simulink model "pfb_coeff_sim"  (R2016b)
settings: Solver=VariableStepAuto  StartTime=0.0  StopTime=8192*0.5  RelTol=1e-3
undefined symbols (not defined in the file): fft_stages
libraries: xbsIndex_r4 x6420, casper_library_misc x5, casper_library_sources x4, xps_library x1, casper_library_delays x1
(part 6 of 36)

== system pfb_coeff_sim/pfb ==
  note: Controls whether there is
      | a shift to the right after
      | multiplication at the
      | respective stage in the
      | fft to prevent
      | overflow.
  note: polyphase FIR and FFT
  shift : Inport
  sync_in : Inport  Port=2
  din0 : Inport  Port=3
  din1 : Inport  Port=4
  en : Inport  Port=5
  Constant : xbsIndex_r4/Constant  const=0  gui_display_data_type=Boolean  arith_type=Boolean  n_bits=16  bin_pt=14  preci_type=Single  exp_width=8  frac_width=24  explicit_period=on  period=1  equ=P=C  opselect=C  inp2=PCIN>>17  opr=+  inp1=P  carry=CIN  dbl_ovrd=off  block_type=constant
  Constant1 : xbsIndex_r4/Constant  const=0  gui_display_data_type=Boolean  arith_type=Boolean  n_bits=16  bin_pt=14  preci_type=Single  exp_width=8  frac_width=24  explicit_period=on  period=1  equ=P=C  opselect=C  inp2=PCIN>>17  opr=+  inp1=P  carry=CIN  dbl_ovrd=off  block_type=constant
  Constant2 : xbsIndex_r4/Constant  const=0  gui_display_data_type=Fixed-point  arith_type=Signed (2's comp)  n_bits=18  bin_pt=17  preci_type=Single  exp_width=8  frac_width=24  explicit_period=on  period=1  equ=P=C  opselect=C  inp2=PCIN>>17  opr=+  inp1=P  carry=CIN  dbl_ovrd=off  block_type=constant
  Constant3 : xbsIndex_r4/Constant  const=0  gui_display_data_type=Fixed-point  arith_type=Unsigned  n_bits=4  bin_pt=0  preci_type=Single  exp_width=8  frac_width=24  explicit_period=on  period=1  equ=P=C  opselect=C  inp2=PCIN>>17  opr=+  inp1=P  carry=CIN  dbl_ovrd=off  block_type=constant
  Constant34 : xbsIndex_r4/Constant  const=0  gui_display_data_type=Fixed-point  arith_type=Unsigned  n_bits=2  bin_pt=0  preci_type=Single  exp_width=8  frac_width=24  explicit_period=on  period=1  equ=P=C  opselect=C  inp2=PCIN>>17  opr=+  inp1=P  carry=CIN  dbl_ovrd=off  block_type=constant
  Gateway Out{1..7,16..17,19,53} (11 alike) : xbsIndex_r4/Gateway Out  inherit_from_input=off  hdl_port=off  rows=1  columns=1  UseAsDAC=off  DACChannel='1'  interface=None  automatic_assignment=on  address_offset=hex2dec('00')  intf_name=''  intf_description=''  timing_constraint=None  locs_specified=off  LOCs={}  io_standard={}  block_type=gatewayout
  Terminator{1..9} (9 alike) : Terminator
  To Workspace16 : ToWorkspace  VariableName=fir_sync_in  SaveFormat=Timeseries  SampleTime=-1
  To Workspace17 : ToWorkspace  VariableName=fir_sync_out  SaveFormat=Timeseries  SampleTime=-1
  To Workspace19 : ToWorkspace  VariableName=fir_dv  SaveFormat=Timeseries  SampleTime=-1
  To Workspace2 : ToWorkspace  VariableName=fir1  SaveFormat=Timeseries  SampleTime=-1
  To Workspace3 : ToWorkspace  VariableName=fir2  SaveFormat=Timeseries  SampleTime=-1
  To Workspace4 : ToWorkspace  VariableName=fir3  SaveFormat=Timeseries  SampleTime=-1
  To Workspace5 : ToWorkspace  VariableName=fir4  SaveFormat=Timeseries  SampleTime=-1
  To Workspace6 : ToWorkspace  VariableName=fir5  SaveFormat=Timeseries  SampleTime=-1
  To Workspace7 : ToWorkspace  VariableName=fir6  SaveFormat=Timeseries  SampleTime=-1
  To Workspace8 : ToWorkspace  VariableName=fir7  SaveFormat=Timeseries  SampleTime=-1
  To Workspace95 : ToWorkspace  VariableName=fir0  SaveFormat=Timeseries  SampleTime=-1
  bus_create3 : Subsystem  AncestorBlock=casper_library_flow_control/bus_create  mask(bus_create){inputNum=4}
      mask prompts: inputNum "Number of inputs:"
      mask init:
      | bus_create_init(gcb,...
      |     'inputNum', inputNum);
  bus_create4 : Subsystem  AncestorBlock=casper_library_flow_control/bus_create  mask(bus_create){inputNum=4}
      mask prompts: inputNum "Number of inputs:"
      mask init:
      | bus_create_init(gcb,...
      |     'inputNum', inputNum);
  bus_expand1 : Subsystem  AncestorBlock=casper_library_flow_control/bus_expand  mask(bus_expand){mode=divisions of equal size, outputNum=8, outputWidth=10, outputBinaryPt=9, outputArithmeticType=1, show_format=off, outputToWorkspace=off, variablePrefix=out, outputToModelAsWell=on}
      mask prompts: outputNum "Number of outputs:"; outputWidth "Output width:"; outputBinaryPt "Output binary point position:"; outputArithmeticType "Output arithmetic type (ufix=0, fix=1, bool=2):"; show_format "Print format string?"; outputToWorkspace "Output to workspace?"; variablePrefix "Variable name prefix:"; outputToModelAsWell "Output to model as well?"
      mask help:
      | Expands a 'bus' made using a bus_create or Xilinx
      | concat block.
      | The input will be divided into the specified number
      | of outputs with the specified arithmetic types.
      | Divisions are made from most significant bit.
      mask init: same as pfb_coeff_sim/bus_expand5
      settings: AttributesFormatString=8 outputs
      mask TypeOptions mode: divisions of equal size | divisions of arbitrary size
      mask Callback mode: bus_expand_callback();
      mask Callback outputWidth: bus_expand_callback();
      mask Callback outputToWorkspace: bus_expand_callback();
  bus_expand2 : Subsystem  AncestorBlock=casper_library_flow_control/bus_expand  mask(bus_expand){mode=divisions of equal size, outputNum=8, outputWidth=10, outputBinaryPt=9, outputArithmeticType=1, show_format=off, outputToWorkspace=off, variablePrefix=out, outputToModelAsWell=on}
      mask prompts: outputNum "Number of outputs:"; outputWidth "Output width:"; outputBinaryPt "Output binary point position:"; outputArithmeticType "Output arithmetic type (ufix=0, fix=1, bool=2):"; show_format "Print format string?"; outputToWorkspace "Output to workspace?"; variablePrefix "Variable name prefix:"; outputToModelAsWell "Output to model as well?"
      mask help:
      | Expands a 'bus' made using a bus_create or Xilinx
      | concat block.
      | The input will be divided into the specified number
      | of outputs with the specified arithmetic types.
      | Divisions are made from most significant bit.
      mask init: same as pfb_coeff_sim/bus_expand5
      settings: AttributesFormatString=8 outputs
      mask TypeOptions mode: divisions of equal size | divisions of arbitrary size
      mask Callback mode: bus_expand_callback();
      mask Callback outputWidth: bus_expand_callback();
      mask Callback outputToWorkspace: bus_expand_callback();
  bus_relational : Subsystem  AncestorBlock=casper_library_bus/bus_relational  mask(bus_relational){n_bits_a=[2 2], bin_pt_a=0, type_a=0, n_bits_b=[2], bin_pt_b=0, type_b=0, en=off, misc=off, mode=a!=b, latency=1}
      mask prompts: n_bits_a "a input bit widths"; bin_pt_a "a input binary points"; type_a "a input type (Unsigned=0, Signed=1)"; n_bits_b "b input bit widths"; bin_pt_b "b input binary points"; type_b "b input type (Unsigned=0, Signed=1)"; en "en port"; misc "misc support"; mode "comparison:"
      mask help: Find the relational product of two busses
      mask init:
      | bus_relational_init(gcb, ...
      |     'n_bits_a', n_bits_a, ...
      |     'bin_pt_a', bin_pt_a, ...
      |     'type_a', type_a, ...
      |     'n_bits_b', n_bits_b, ...
      |     'bin_pt_b', bin_pt_b, ...
      |     'type_b', type_b, ...
      |     'en', en, ...
      |     'misc', misc, ...
      |     'mode', mode, ...
      |     'latency', latency);
      mask TypeOptions mode: a=b | a!=b | a<b | a>b | a<=b | a>=b
  pfb_fir_generic : Subsystem  Tag=casper:pfb_fir_generic  AncestorBlock=casper_library_pfbs/pfb_fir_generic  mask(pfb_fir_generic){n_streams=1, PFBSize=n_bits_fft, TotalTaps=n_taps, WindowType=hann, n_inputs=3, BitWidthIn=10, BitWidthOut=18, CoeffBitWidth=18, complex=off, async=on, add_latency=4, mult_latency=3, bram_latency=3, fan_latency=6, conv_latency=4, quantization=Round  (unbiased: Even Values), fwidth=1, coeffs_bram_optimization=Speed, delays_bram_optimization=Speed}
      mask prompts: n_streams "Number input streams?"; PFBSize "Size of PFB: (2^? pnts)"; TotalTaps "Total Number of Taps:"; WindowType "Windowing Function:"; n_inputs "Number of Simultaneous Inputs: (2^?)"; BitWidthIn "Input Bitwidth:"; BitWidthOut "Output Bitwidth:"; CoeffBitWidth "Coefficient Bitwidth:"; complex "Complex data inputs"; async "Asynchronous operation"; add_latency "Add Latency"; mult_latency "Mult Latency"; bram_latency "BRAM Latency"; fan_latency "Fanout Latency"; conv_latency "Convert latency"; quantization "Quantization Behavior"; fwidth "Bin Width Scaling (normal=1)"; coeffs_bram_optimization "Coefficient BRAMs optimization"; delays_bram_optimization "Delay BRAMs optimization"
      mask init:
      | pfb_fir_generic_init(gcb, ...
      |     'n_streams', n_streams, ...
      |     'PFBSize', PFBSize, ...
      |     'TotalTaps', TotalTaps, ...
      |     'WindowType', WindowType, ...
      |     'n_inputs', n_inputs, ...
      |     'complex', complex, ...
      |     'BitWidthIn', BitWidthIn, ...
      |     'BitWidthOut', BitWidthOut, ...
      |     'CoeffBitWidth', CoeffBitWidth, ...
      |     'async', async, ...
      |     'add_latency', add_latency, ...
      |     'mult_latency', mult_latency, ...
      |     'bram_latency', bram_latency, ...
      |     'fan_latency', fan_latency, ...
      |     'conv_latency', conv_latency, ...
      |     'quantization', quantization, ...
      |     'fwidth', fwidth, ...
      |     'coeffs_bram_optimization', coeffs_bram_optimization, ...
      |     'delays_bram_optimization', delays_bram_optimization);
      mask Callback TotalTaps:
      | %num_taps = eval(get_param(gcb, 'TotalTaps'));
      | %old_vec = eval(get_param(gcb, 'mult_spec'));
      | 
      | %vec = 2.*ones(1,num_taps);
      | %old_size = length(old_vec);
      | 
      | %if(old_size <= num_taps),
      | %   new_size = old_size;
      | %else,
      | %    new_size = num_taps;
      | %end
      | 
      | %for n = 1:new_size, vec(n) = old_vec(n); end
      | %set_param(gcb, 'mult_spec', mat2str(vec));
      mask TypeOptions WindowType: bartlett | barthannwin | blackman | blackmanharris | bohamwin | chebwin | flattopwin | gausswin | hamming | hann | kaiser | nuttallwin | parzenwin | rectwin | tukeywin | triang | userwindow
      mask TypeOptions quantization: Truncate | Round  (unbiased: +/- Inf) | Round  (unbiased: Even Values)
      mask Callback fwidth:
      | %num_taps = eval(get_param(gcb, 'TotalTaps'));
      | %old_vec = eval(get_param(gcb, 'mult_spec'));
      | 
      | %vec = 2.*ones(1,num_taps);
      | %old_size = length(old_vec);
      | 
      | %if(old_size <= num_taps),
      | %    new_size = old_size;
      | %else,
      | %    new_size = num_taps;
      | %end
      | 
      | %for n = 1:new_size, vec(n) = old_vec(n); end
      | %set_param(gcb, 'mult_spec', mat2str(vec));
      mask TypeOptions coeffs_bram_optimization: Area | Speed
      mask TypeOptions delays_bram_optimization: Area | Speed
  pipeline11 : Subsystem  AncestorBlock=casper_library_delays/pipeline  mask(pipeline){latency=2}
      mask help:
      | An explicitly laid-out delay line to avoid mapping to SRL16s
      | for use in pipelining to help achieve timing closure.
      mask init:
      | pipeline_init(gcb,'latency',latency);
      settings: AttributesFormatString=Latency = %<latency>
      mask Display:
      | port_label('input', 1, 'd');
      | port_label('output', 1, 'q');
      | disp(['Z^-', num2str(latency)]);
  pipeline12 : Subsystem  AncestorBlock=casper_library_delays/pipeline  mask(pipeline){latency=2}
      mask help:
      | An explicitly laid-out delay line to avoid mapping to SRL16s
      | for use in pipelining to help achieve timing closure.
      mask init:
      | pipeline_init(gcb,'latency',latency);
      settings: AttributesFormatString=Latency = %<latency>
      mask Display:
      | port_label('input', 1, 'd');
      | port_label('output', 1, 'q');
      | disp(['Z^-', num2str(latency)]);
  pipeline13 : Subsystem  AncestorBlock=casper_library_delays/pipeline  mask(pipeline){latency=2}
      mask help:
      | An explicitly laid-out delay line to avoid mapping to SRL16s
      | for use in pipelining to help achieve timing closure.
      mask init:
      | pipeline_init(gcb,'latency',latency);
      settings: AttributesFormatString=Latency = %<latency>
      mask Display:
      | port_label('input', 1, 'd');
      | port_label('output', 1, 'q');
      | disp(['Z^-', num2str(latency)]);
  pipeline14 : Subsystem  AncestorBlock=casper_library_delays/pipeline  mask(pipeline){latency=2}
      mask help:
      | An explicitly laid-out delay line to avoid mapping to SRL16s
      | for use in pipelining to help achieve timing closure.
      mask init:
      | pipeline_init(gcb,'latency',latency);
      settings: AttributesFormatString=Latency = %<latency>
      mask Display:
      | port_label('input', 1, 'd');
      | port_label('output', 1, 'q');
      | disp(['Z^-', num2str(latency)]);
  pipeline24 : Subsystem  AncestorBlock=casper_library_delays/pipeline  mask(pipeline){latency=2}
      mask help:
      | An explicitly laid-out delay line to avoid mapping to SRL16s
      | for use in pipelining to help achieve timing closure.
      mask init:
      | pipeline_init(gcb,'latency',latency);
      settings: AttributesFormatString=Latency = %<latency>
      mask Display:
      | port_label('input', 1, 'd');
      | port_label('output', 1, 'q');
      | disp(['Z^-', num2str(latency)]);
  pipeline26 : Subsystem  AncestorBlock=casper_library_delays/pipeline  mask(pipeline){latency=2}
      mask help:
      | An explicitly laid-out delay line to avoid mapping to SRL16s
      | for use in pipelining to help achieve timing closure.
      mask init:
      | pipeline_init(gcb,'latency',latency);
      settings: AttributesFormatString=Latency = %<latency>
      mask Display:
      | port_label('input', 1, 'd');
      | port_label('output', 1, 'q');
      | disp(['Z^-', num2str(latency)]);
  pipeline34 : Subsystem  AncestorBlock=casper_library_delays/pipeline  mask(pipeline){latency=2}
      mask help:
      | An explicitly laid-out delay line to avoid mapping to SRL16s
      | for use in pipelining to help achieve timing closure.
      mask init:
      | pipeline_init(gcb,'latency',latency);
      settings: AttributesFormatString=Latency = %<latency>
      mask Display:
      | port_label('input', 1, 'd');
      | port_label('output', 1, 'q');
      | disp(['Z^-', num2str(latency)]);
  pipeline35 : Subsystem  AncestorBlock=casper_library_delays/pipeline  mask(pipeline){latency=2}
      mask help:
      | An explicitly laid-out delay line to avoid mapping to SRL16s
      | for use in pipelining to help achieve timing closure.
      mask init:
      | pipeline_init(gcb,'latency',latency);
      settings: AttributesFormatString=Latency = %<latency>
      mask Display:
      | port_label('input', 1, 'd');
      | port_label('output', 1, 'q');
      | disp(['Z^-', num2str(latency)]);
  pipeline36 : Subsystem  AncestorBlock=casper_library_delays/pipeline  mask(pipeline){latency=2}
      mask help:
      | An explicitly laid-out delay line to avoid mapping to SRL16s
      | for use in pipelining to help achieve timing closure.
      mask init:
      | pipeline_init(gcb,'latency',latency);
      settings: AttributesFormatString=Latency = %<latency>
      mask Display:
      | port_label('input', 1, 'd');
      | port_label('output', 1, 'q');
      | disp(['Z^-', num2str(latency)]);
  pipeline37 : Subsystem  AncestorBlock=casper_library_delays/pipeline  mask(pipeline){latency=2}
      mask help:
      | An explicitly laid-out delay line to avoid mapping to SRL16s
      | for use in pipelining to help achieve timing closure.
      mask init:
      | pipeline_init(gcb,'latency',latency);
      settings: AttributesFormatString=Latency = %<latency>
      mask Display:
      | port_label('input', 1, 'd');
      | port_label('output', 1, 'q');
      | disp(['Z^-', num2str(latency)]);
  pipeline38 : Subsystem  AncestorBlock=casper_library_delays/pipeline  mask(pipeline){latency=2}
      mask help:
      | An explicitly laid-out delay line to avoid mapping to SRL16s
      | for use in pipelining to help achieve timing closure.
      mask init:
      | pipeline_init(gcb,'latency',latency);
      settings: AttributesFormatString=Latency = %<latency>
      mask Display:
      | port_label('input', 1, 'd');
      | port_label('output', 1, 'q');
      | disp(['Z^-', num2str(latency)]);
  pipeline39 : Subsystem  AncestorBlock=casper_library_delays/pipeline  mask(pipeline){latency=2}
      mask help:
      | An explicitly laid-out delay line to avoid mapping to SRL16s
      | for use in pipelining to help achieve timing closure.
      mask init:
      | pipeline_init(gcb,'latency',latency);
      settings: AttributesFormatString=Latency = %<latency>
      mask Display:
      | port_label('input', 1, 'd');
      | port_label('output', 1, 'q');
      | disp(['Z^-', num2str(latency)]);
  pipeline40 : Subsystem  AncestorBlock=casper_library_delays/pipeline  mask(pipeline){latency=2}
      mask help:
      | An explicitly laid-out delay line to avoid mapping to SRL16s
      | for use in pipelining to help achieve timing closure.
      mask init:
      | pipeline_init(gcb,'latency',latency);
      settings: AttributesFormatString=Latency = %<latency>
      mask Display:
      | port_label('input', 1, 'd');
      | port_label('output', 1, 'q');
      | disp(['Z^-', num2str(latency)]);
  pipeline41 : Subsystem  AncestorBlock=casper_library_delays/pipeline  mask(pipeline){latency=2}
      mask help:
      | An explicitly laid-out delay line to avoid mapping to SRL16s
      | for use in pipelining to help achieve timing closure.
      mask init:
      | pipeline_init(gcb,'latency',latency);
      settings: AttributesFormatString=Latency = %<latency>
      mask Display:
      | port_label('input', 1, 'd');
      | port_label('output', 1, 'q');
      | disp(['Z^-', num2str(latency)]);
  pipeline9 : Subsystem  AncestorBlock=casper_library_delays/pipeline  mask(pipeline){latency=2}
      mask help:
      | An explicitly laid-out delay line to avoid mapping to SRL16s
      | for use in pipelining to help achieve timing closure.
      mask init:
      | pipeline_init(gcb,'latency',latency);
      settings: AttributesFormatString=Latency = %<latency>
      mask Display:
      | port_label('input', 1, 'd');
      | port_label('output', 1, 'q');
      | disp(['Z^-', num2str(latency)]);
  sync_out : Outport
  dout0 : Outport  Port=2
  dout1 : Outport  Port=3
  dvalid : Outport  Port=4
  of : Outport  Port=5
  wires:
  bus_relational/1(a!=b) -> of/1
  Constant34/1 -> bus_relational/2(b)
  pipeline9/1(q) -> bus_relational/1(a)
  sync_in/1 -> pipeline11/1(d)
  din0/1 -> pipeline12/1(d)
  din1/1 -> pipeline13/1(d)
  en/1 -> pipeline14/1(d)
  Constant2/1 -> pipeline35/1(d), pipeline36/1(d), pipeline37/1(d), pipeline38/1(d), pipeline39/1(d), pipeline40/1(d), pipeline41/1(d), pipeline34/1(d)
  pipeline12/1(q) -> bus_expand1/1(bus_in)
  pipeline13/1(q) -> bus_expand2/1(bus_in)
  pipeline34/1(q) -> bus_create3/1(in1)
  pipeline35/1(q) -> bus_create3/2(in2)
  pipeline38/1(q) -> bus_create4/1(in1)
  pipeline36/1(q) -> bus_create3/3(in3)
  pipeline37/1(q) -> bus_create3/4(in4)
  pipeline39/1(q) -> bus_create4/2(in2)
  pipeline40/1(q) -> bus_create4/3(in3)
  pipeline41/1(q) -> bus_create4/4(in4)
  bus_expand1/6(out3) -> pfb_fir_generic/7(pol0_in5)
  bus_expand1/5(out4) -> pfb_fir_generic/6(pol0_in4)
  bus_expand1/1(msb_out8) -> pfb_fir_generic/2(pol0_in0)
  bus_expand1/8(lsb_out1) -> pfb_fir_generic/9(pol0_in7)
  bus_expand1/2(out7) -> pfb_fir_generic/3(pol0_in1)
  bus_expand1/4(out5) -> pfb_fir_generic/5(pol0_in3)
  bus_expand1/3(out6) -> pfb_fir_generic/4(pol0_in2)
  bus_expand1/7(out2) -> pfb_fir_generic/8(pol0_in6)
  Constant/1 -> pipeline24/1(d)
  bus_create3/1(bus_out) -> dout0/1
  bus_create4/1(bus_out) -> dout1/1
  Constant1/1 -> pipeline26/1(d)
  pfb_fir_generic/10(dvalid) -> Gateway Out19/1
  pfb_fir_generic/9(pol0_out7) -> Gateway Out7/1
  pfb_fir_generic/8(pol0_out6) -> Gateway Out6/1
  pfb_fir_generic/7(pol0_out5) -> Gateway Out5/1
  pfb_fir_generic/6(pol0_out4) -> Gateway Out4/1
  pfb_fir_generic/5(pol0_out3) -> Gateway Out3/1
  pfb_fir_generic/3(pol0_out1) -> Gateway Out1/1
  pfb_fir_generic/2(pol0_out0) -> Gateway Out53/1
  pfb_fir_generic/1(sync_out) -> Gateway Out17/1
  pipeline24/1(q) -> sync_out/1
  pipeline26/1(q) -> dvalid/1
  Gateway Out53/1 -> To Workspace95/1
  Gateway Out1/1 -> To Workspace2/1
  Gateway Out2/1 -> To Workspace3/1
  Gateway Out3/1 -> To Workspace4/1
  Gateway Out4/1 -> To Workspace5/1
  Gateway Out5/1 -> To Workspace6/1
  Gateway Out6/1 -> To Workspace7/1
  Gateway Out7/1 -> To Workspace8/1
  pfb_fir_generic/4(pol0_out2) -> Gateway Out2/1
  pipeline11/1(q) -> pfb_fir_generic/1(sync), Gateway Out16/1
  Gateway Out16/1 -> To Workspace16/1
  Gateway Out17/1 -> To Workspace17/1
  pipeline14/1(q) -> pfb_fir_generic/10(en)
  Gateway Out19/1 -> To Workspace19/1
  Constant3/1 -> pipeline9/1(d)
  shift/1 -> Terminator8/1
  bus_expand2/1(msb_out8) -> Terminator1/1
  bus_expand2/2(out7) -> Terminator2/1
  bus_expand2/3(out6) -> Terminator3/1
  bus_expand2/4(out5) -> Terminator4/1
  bus_expand2/5(out4) -> Terminator5/1
  bus_expand2/6(out3) -> Terminator6/1
  bus_expand2/7(out2) -> Terminator7/1
  bus_expand2/8(lsb_out1) -> Terminator9/1

== system pfb_coeff_sim/pfb_of ==
  out_reg : Inport
  assert_reg : xbsIndex_r4/Assert  assert_type=on  type_source=Explicitly  gui_display_data_type=Fixed-point  arith_type=Unsigned  n_bits=2  bin_pt=0  preci_type=Single  exp_width=8  frac_width=24  assert_rate=off  rate_source=Explicitly  period=1  output_port=on  block_type=assert
  cast_gw : xbsIndex_r4/Convert  gui_display_data_type=Fixed-point  arith_type=Unsigned  n_bits=32  bin_pt=0  float_type=Single  exp_bits=8  fraction_bits=24  quantization=Truncate  overflow=Wrap  en=off  latency=1  pipeline=off  dbl_ovrd=off  block_type=convert
  io_delay : xbsIndex_r4/Delay  rst=off  infoeditControl=Selection of Reset will increase slice count due to use of real FFs and instead of SRLs  en=off  latency=0  reg_retiming=on  dbl_ovrd=off  block_type=delay
      settings: infoedit=Hardware notes: A delay line is a chain, each link of which is an SRL16 or SRL32 followed by a flip-flop.
  pfb_coeff_sim_pfb_of_user_data_in : xbsIndex_r4/Gateway Out  inherit_from_input=off  hdl_port=on  rows=1  columns=1  UseAsDAC=off  DACChannel='1'  interface=None  automatic_assignment=on  address_offset=hex2dec('00')  intf_name=''  intf_description=''  timing_constraint=None  locs_specified=off  LOCs={}  io_standard={}  block_type=gatewayout
  reint1 : xbsIndex_r4/Reinterpret  force_arith_type=on  arith_type=Unsigned  force_bin_pt=on  bin_pt=0  block_type=reinterpret
  sim_out : Outport
  wires:
  io_delay/1 -> cast_gw/1
  cast_gw/1 -> pfb_coeff_sim_pfb_of_user_data_in/1
  pfb_coeff_sim_pfb_of_user_data_in/1 -> sim_out/1
  out_reg/1 -> assert_reg/1
  assert_reg/1 -> reint1/1
  reint1/1 -> io_delay/1

== system pfb_coeff_sim/pfbin_sync_count ==
  out_reg : Inport
  assert_reg : xbsIndex_r4/Assert  assert_type=on  type_source=Explicitly  gui_display_data_type=Fixed-point  arith_type=Unsigned  n_bits=32  bin_pt=0  preci_type=Single  exp_width=8  frac_width=24  assert_rate=off  rate_source=Explicitly  period=1  output_port=on  block_type=assert
  cast_gw : xbsIndex_r4/Convert  gui_display_data_type=Fixed-point  arith_type=Unsigned  n_bits=32  bin_pt=0  float_type=Single  exp_bits=8  fraction_bits=24  quantization=Truncate  overflow=Wrap  en=off  latency=1  pipeline=off  dbl_ovrd=off  block_type=convert
  io_delay : xbsIndex_r4/Delay  rst=off  infoeditControl=Selection of Reset will increase slice count due to use of real FFs and instead of SRLs  en=off  latency=0  reg_retiming=on  dbl_ovrd=off  block_type=delay
      settings: infoedit=Hardware notes: A delay line is a chain, each link of which is an SRL16 or SRL32 followed by a flip-flop.
  pfb_coeff_sim_pfbin_sync_count_user_data_in : xbsIndex_r4/Gateway Out  inherit_from_input=off  hdl_port=on  rows=1  columns=1  UseAsDAC=off  DACChannel='1'  interface=None  automatic_assignment=on  address_offset=hex2dec('00')  intf_name=''  intf_description=''  timing_constraint=None  locs_specified=off  LOCs={}  io_standard={}  block_type=gatewayout
  reint1 : xbsIndex_r4/Reinterpret  force_arith_type=on  arith_type=Unsigned  force_bin_pt=on  bin_pt=0  block_type=reinterpret
  sim_out : Outport
  wires:
  io_delay/1 -> cast_gw/1
  cast_gw/1 -> pfb_coeff_sim_pfbin_sync_count_user_data_in/1
  pfb_coeff_sim_pfbin_sync_count_user_data_in/1 -> sim_out/1
  out_reg/1 -> assert_reg/1
  assert_reg/1 -> reint1/1
  reint1/1 -> io_delay/1

== system pfb_coeff_sim/pfbout_sync_count ==
  out_reg : Inport
  assert_reg : xbsIndex_r4/Assert  assert_type=on  type_source=Explicitly  gui_display_data_type=Fixed-point  arith_type=Unsigned  n_bits=32  bin_pt=0  preci_type=Single  exp_width=8  frac_width=24  assert_rate=off  rate_source=Explicitly  period=1  output_port=on  block_type=assert
  cast_gw : xbsIndex_r4/Convert  gui_display_data_type=Fixed-point  arith_type=Unsigned  n_bits=32  bin_pt=0  float_type=Single  exp_bits=8  fraction_bits=24  quantization=Truncate  overflow=Wrap  en=off  latency=1  pipeline=off  dbl_ovrd=off  block_type=convert
  io_delay : xbsIndex_r4/Delay  rst=off  infoeditControl=Selection of Reset will increase slice count due to use of real FFs and instead of SRLs  en=off  latency=0  reg_retiming=on  dbl_ovrd=off  block_type=delay
      settings: infoedit=Hardware notes: A delay line is a chain, each link of which is an SRL16 or SRL32 followed by a flip-flop.
  pfb_coeff_sim_pfbout_sync_count_user_data_in : xbsIndex_r4/Gateway Out  inherit_from_input=off  hdl_port=on  rows=1  columns=1  UseAsDAC=off  DACChannel='1'  interface=None  automatic_assignment=on  address_offset=hex2dec('00')  intf_name=''  intf_description=''  timing_constraint=None  locs_specified=off  LOCs={}  io_standard={}  block_type=gatewayout
  reint1 : xbsIndex_r4/Reinterpret  force_arith_type=on  arith_type=Unsigned  force_bin_pt=on  bin_pt=0  block_type=reinterpret
  sim_out : Outport
  wires:
  io_delay/1 -> cast_gw/1
  cast_gw/1 -> pfb_coeff_sim_pfbout_sync_count_user_data_in/1
  pfb_coeff_sim_pfbout_sync_count_user_data_in/1 -> sim_out/1
  out_reg/1 -> assert_reg/1
  assert_reg/1 -> reint1/1
  reint1/1 -> io_delay/1

== system pfb_coeff_sim/pipeline1 ==
  d : Inport
  Register0 : xbsIndex_r4/Register  init=0  rst=off  en=off  dbl_ovrd=off  block_type=register
      settings: block_version=11.4
  Register1 : xbsIndex_r4/Register  init=0  rst=off  en=off  dbl_ovrd=off  block_type=register
      settings: block_version=11.4
  q : Outport
  wires:
  Register0/1 -> Register1/1
  d/1 -> Register0/1
  Register1/1 -> q/1

== system pfb_coeff_sim/pipeline10 ==
  d : Inport
  Register0 : xbsIndex_r4/Register  init=0  rst=off  en=off  dbl_ovrd=off  block_type=register
      settings: block_version=11.4
  Register1 : xbsIndex_r4/Register  init=0  rst=off  en=off  dbl_ovrd=off  block_type=register
      settings: block_version=11.4
  q : Outport
  wires:
  Register1/1 -> q/1
  d/1 -> Register0/1
  Register0/1 -> Register1/1

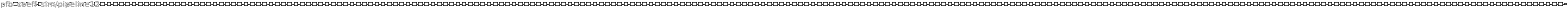
== system pfb_coeff_sim/pipeline12 ==
  d : Inport
  Register{0..249} (250 alike) : xbsIndex_r4/Register  init=0  rst=off  en=off  dbl_ovrd=off  block_type=register
      Register0 settings: block_version=11.4
      Register1 settings: block_version=11.4
  q : Outport
  wires:
  Register249/1 -> q/1
  d/1 -> Register0/1
  Register248/1 -> Register249/1
  Register247/1 -> Register248/1
  Register246/1 -> Register247/1
  Register245/1 -> Register246/1
  Register244/1 -> Register245/1
  Register243/1 -> Register244/1
  Register242/1 -> Register243/1
  Register241/1 -> Register242/1
  Register240/1 -> Register241/1
  Register239/1 -> Register240/1
  Register238/1 -> Register239/1
  Register237/1 -> Register238/1
  Register236/1 -> Register237/1
  Register235/1 -> Register236/1
  Register234/1 -> Register235/1
  Register233/1 -> Register234/1
  Register232/1 -> Register233/1
  Register231/1 -> Register232/1
  Register230/1 -> Register231/1
  Register229/1 -> Register230/1
  Register228/1 -> Register229/1
  Register227/1 -> Register228/1
  Register226/1 -> Register227/1
  Register225/1 -> Register226/1
  Register224/1 -> Register225/1
  Register223/1 -> Register224/1
  Register222/1 -> Register223/1
  Register221/1 -> Register222/1
  Register220/1 -> Register221/1
  Register219/1 -> Register220/1
  Register218/1 -> Register219/1
  Register217/1 -> Register218/1
  Register216/1 -> Register217/1
  Register215/1 -> Register216/1
  Register214/1 -> Register215/1
  Register213/1 -> Register214/1
  Register212/1 -> Register213/1
  Register211/1 -> Register212/1
  Register210/1 -> Register211/1
  Register209/1 -> Register210/1
  Register208/1 -> Register209/1
  Register207/1 -> Register208/1
  Register206/1 -> Register207/1
  Register205/1 -> Register206/1
  Register204/1 -> Register205/1
  Register203/1 -> Register204/1
  Register202/1 -> Register203/1
  Register201/1 -> Register202/1
  Register200/1 -> Register201/1
  Register199/1 -> Register200/1
  Register198/1 -> Register199/1
  Register197/1 -> Register198/1
  Register196/1 -> Register197/1
  Register195/1 -> Register196/1
  Register194/1 -> Register195/1
  Register193/1 -> Register194/1
  Register192/1 -> Register193/1
  Register191/1 -> Register192/1
  Register190/1 -> Register191/1
  Register189/1 -> Register190/1
  Register188/1 -> Register189/1
  Register187/1 -> Register188/1
  Register186/1 -> Register187/1
  Register185/1 -> Register186/1
  Register184/1 -> Register185/1
  Register183/1 -> Register184/1
  Register182/1 -> Register183/1
  Register181/1 -> Register182/1
  Register180/1 -> Register181/1
  Register179/1 -> Register180/1
  Register178/1 -> Register179/1
  Register177/1 -> Register178/1
  Register176/1 -> Register177/1
  Register175/1 -> Register176/1
  Register174/1 -> Register175/1
  Register173/1 -> Register174/1
  Register172/1 -> Register173/1
  Register171/1 -> Register172/1
  Register170/1 -> Register171/1
  Register169/1 -> Register170/1
  Register168/1 -> Register169/1
  Register167/1 -> Register168/1
  Register166/1 -> Register167/1
  Register165/1 -> Register166/1
  Register164/1 -> Register165/1
  Register163/1 -> Register164/1
  Register162/1 -> Register163/1
  Register161/1 -> Register162/1
  Register160/1 -> Register161/1
  Register159/1 -> Register160/1
  Register158/1 -> Register159/1
  Register157/1 -> Register158/1
  Register156/1 -> Register157/1
  Register155/1 -> Register156/1
  Register154/1 -> Register155/1
  Register153/1 -> Register154/1
  Register152/1 -> Register153/1
  Register151/1 -> Register152/1
  Register150/1 -> Register151/1
  Register149/1 -> Register150/1
  Register148/1 -> Register149/1
  Register147/1 -> Register148/1
  Register146/1 -> Register147/1
  Register145/1 -> Register146/1
  Register144/1 -> Register145/1
  Register143/1 -> Register144/1
  Register142/1 -> Register143/1
  Register141/1 -> Register142/1
  Register140/1 -> Register141/1
  Register139/1 -> Register140/1
  Register138/1 -> Register139/1
  Register137/1 -> Register138/1
  Register136/1 -> Register137/1
  Register135/1 -> Register136/1
  Register134/1 -> Register135/1
  Register133/1 -> Register134/1
  Register132/1 -> Register133/1
  Register131/1 -> Register132/1
  Register130/1 -> Register131/1
  Register129/1 -> Register130/1
  Register128/1 -> Register129/1
  Register127/1 -> Register128/1
  Register126/1 -> Register127/1
  Register125/1 -> Register126/1
  Register124/1 -> Register125/1
  Register123/1 -> Register124/1
  Register122/1 -> Register123/1
  Register121/1 -> Register122/1
  Register120/1 -> Register121/1
  Register119/1 -> Register120/1
  Register118/1 -> Register119/1
  Register117/1 -> Register118/1
  Register116/1 -> Register117/1
  Register115/1 -> Register116/1
  Register114/1 -> Register115/1
  Register113/1 -> Register114/1
  Register112/1 -> Register113/1
  Register111/1 -> Register112/1
  Register110/1 -> Register111/1
  Register109/1 -> Register110/1
  Register108/1 -> Register109/1
  Register107/1 -> Register108/1
  Register106/1 -> Register107/1
  Register105/1 -> Register106/1
  Register104/1 -> Register105/1
  Register103/1 -> Register104/1
  Register102/1 -> Register103/1
  Register101/1 -> Register102/1
  Register100/1 -> Register101/1
  Register99/1 -> Register100/1
  Register98/1 -> Register99/1
  Register97/1 -> Register98/1
  Register96/1 -> Register97/1
  Register95/1 -> Register96/1
  Register94/1 -> Register95/1
  Register93/1 -> Register94/1
  Register92/1 -> Register93/1
  Register91/1 -> Register92/1
  Register90/1 -> Register91/1
  Register89/1 -> Register90/1
  Register88/1 -> Register89/1
  Register87/1 -> Register88/1
  Register86/1 -> Register87/1
  Register85/1 -> Register86/1
  Register84/1 -> Register85/1
  Register83/1 -> Register84/1
  Register82/1 -> Register83/1
  Register81/1 -> Register82/1
  Register80/1 -> Register81/1
  Register79/1 -> Register80/1
  Register78/1 -> Register79/1
  Register77/1 -> Register78/1
  Register76/1 -> Register77/1
  Register75/1 -> Register76/1
  Register74/1 -> Register75/1
  Register73/1 -> Register74/1
  Register72/1 -> Register73/1
  Register71/1 -> Register72/1
  Register70/1 -> Register71/1
  Register69/1 -> Register70/1
  Register68/1 -> Register69/1
  Register67/1 -> Register68/1
  Register66/1 -> Register67/1
  Register65/1 -> Register66/1
  Register64/1 -> Register65/1
  Register63/1 -> Register64/1
  Register62/1 -> Register63/1
  Register61/1 -> Register62/1
  Register60/1 -> Register61/1
  Register59/1 -> Register60/1
  Register58/1 -> Register59/1
  Register57/1 -> Register58/1
  Register56/1 -> Register57/1
  Register55/1 -> Register56/1
  Register54/1 -> Register55/1
  Register53/1 -> Register54/1
  Register52/1 -> Register53/1
  Register51/1 -> Register52/1
  Register50/1 -> Register51/1
  Register49/1 -> Register50/1
  Register48/1 -> Register49/1
  Register47/1 -> Register48/1
  Register46/1 -> Register47/1
  Register45/1 -> Register46/1
  Register44/1 -> Register45/1
  Register43/1 -> Register44/1
  Register42/1 -> Register43/1
  Register41/1 -> Register42/1
  Register40/1 -> Register41/1
  Register39/1 -> Register40/1
  Register38/1 -> Register39/1
  Register37/1 -> Register38/1
  Register36/1 -> Register37/1
  Register35/1 -> Register36/1
  Register34/1 -> Register35/1
  Register33/1 -> Register34/1
  Register32/1 -> Register33/1
  Register31/1 -> Register32/1
  Register30/1 -> Register31/1
  Register29/1 -> Register30/1
  Register28/1 -> Register29/1
  Register27/1 -> Register28/1
  Register26/1 -> Register27/1
  Register25/1 -> Register26/1
  Register24/1 -> Register25/1
  Register23/1 -> Register24/1
  Register22/1 -> Register23/1
  Register21/1 -> Register22/1
  Register20/1 -> Register21/1
  Register19/1 -> Register20/1
  Register18/1 -> Register19/1
  Register17/1 -> Register18/1
  Register16/1 -> Register17/1
  Register15/1 -> Register16/1
  Register14/1 -> Register15/1
  Register13/1 -> Register14/1
  Register12/1 -> Register13/1
  Register11/1 -> Register12/1
  Register10/1 -> Register11/1
  Register9/1 -> Register10/1
  Register8/1 -> Register9/1
  Register7/1 -> Register8/1
  Register6/1 -> Register7/1
  Register5/1 -> Register6/1
  Register4/1 -> Register5/1
  Register3/1 -> Register4/1
  Register2/1 -> Register3/1
  Register1/1 -> Register2/1
  Register0/1 -> Register1/1

== system pfb_coeff_sim/pipeline180 ==
  d : Inport
  Register0 : xbsIndex_r4/Register  init=0  rst=off  en=off  dbl_ovrd=off  block_type=register
      settings: block_version=11.4
  Register1 : xbsIndex_r4/Register  init=0  rst=off  en=off  dbl_ovrd=off  block_type=register
      settings: block_version=11.4
  q : Outport
  wires:
  Register0/1 -> Register1/1
  d/1 -> Register0/1
  Register1/1 -> q/1

== system pfb_coeff_sim/pipeline181 ==
  d : Inport
  Register0 : xbsIndex_r4/Register  init=0  rst=off  en=off  dbl_ovrd=off  block_type=register
      settings: block_version=11.4
  Register1 : xbsIndex_r4/Register  init=0  rst=off  en=off  dbl_ovrd=off  block_type=register
      settings: block_version=11.4
  q : Outport
  wires:
  Register1/1 -> q/1
  d/1 -> Register0/1
  Register0/1 -> Register1/1

== system pfb_coeff_sim/pipeline182 ==
  d : Inport
  Register0 : xbsIndex_r4/Register  init=0  rst=off  en=off  dbl_ovrd=off  block_type=register
      settings: block_version=11.4
  Register1 : xbsIndex_r4/Register  init=0  rst=off  en=off  dbl_ovrd=off  block_type=register
      settings: block_version=11.4
  q : Outport
  wires:
  Register0/1 -> Register1/1
  d/1 -> Register0/1
  Register1/1 -> q/1

== system pfb_coeff_sim/pipeline198 ==
  d : Inport
  Register0 : xbsIndex_r4/Register  init=0  rst=off  en=off  dbl_ovrd=off  block_type=register
      settings: block_version=11.4
  Register1 : xbsIndex_r4/Register  init=0  rst=off  en=off  dbl_ovrd=off  block_type=register
      settings: block_version=11.4
  q : Outport
  wires:
  Register1/1 -> q/1
  d/1 -> Register0/1
  Register0/1 -> Register1/1

== system pfb_coeff_sim/pipeline2 ==
  d : Inport
  Register0 : xbsIndex_r4/Register  init=0  rst=off  en=off  dbl_ovrd=off  block_type=register
      settings: block_version=11.4
  Register1 : xbsIndex_r4/Register  init=0  rst=off  en=off  dbl_ovrd=off  block_type=register
      settings: block_version=11.4
  q : Outport
  wires:
  Register1/1 -> q/1
  d/1 -> Register0/1
  Register0/1 -> Register1/1

== system pfb_coeff_sim/pipeline3 ==
  d : Inport
  Register0 : xbsIndex_r4/Register  init=0  rst=off  en=off  dbl_ovrd=off  block_type=register
      settings: block_version=11.4
  Register1 : xbsIndex_r4/Register  init=0  rst=off  en=off  dbl_ovrd=off  block_type=register
      settings: block_version=11.4
  q : Outport
  wires:
  Register0/1 -> Register1/1
  d/1 -> Register0/1
  Register1/1 -> q/1

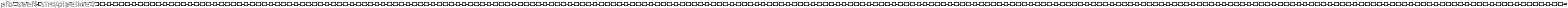
== system pfb_coeff_sim/pipeline4 ==
  d : Inport
  Register{0..249} (250 alike) : xbsIndex_r4/Register  init=0  rst=off  en=off  dbl_ovrd=off  block_type=register
      Register0 settings: block_version=11.4
      Register1 settings: block_version=11.4
  q : Outport
  wires:
  Register0/1 -> Register1/1
  Register1/1 -> Register2/1
  Register2/1 -> Register3/1
  Register3/1 -> Register4/1
  Register4/1 -> Register5/1
  Register5/1 -> Register6/1
  Register6/1 -> Register7/1
  Register7/1 -> Register8/1
  Register8/1 -> Register9/1
  Register9/1 -> Register10/1
  Register10/1 -> Register11/1
  Register11/1 -> Register12/1
  Register12/1 -> Register13/1
  Register13/1 -> Register14/1
  Register14/1 -> Register15/1
  Register15/1 -> Register16/1
  Register16/1 -> Register17/1
  Register17/1 -> Register18/1
  Register18/1 -> Register19/1
  Register19/1 -> Register20/1
  Register20/1 -> Register21/1
  Register21/1 -> Register22/1
  Register22/1 -> Register23/1
  Register23/1 -> Register24/1
  Register24/1 -> Register25/1
  Register25/1 -> Register26/1
  Register26/1 -> Register27/1
  Register27/1 -> Register28/1
  Register28/1 -> Register29/1
  Register29/1 -> Register30/1
  Register30/1 -> Register31/1
  Register31/1 -> Register32/1
  Register32/1 -> Register33/1
  Register33/1 -> Register34/1
  Register34/1 -> Register35/1
  Register35/1 -> Register36/1
  Register36/1 -> Register37/1
  Register37/1 -> Register38/1
  Register38/1 -> Register39/1
  Register39/1 -> Register40/1
  Register40/1 -> Register41/1
  Register41/1 -> Register42/1
  Register42/1 -> Register43/1
  Register43/1 -> Register44/1
  Register44/1 -> Register45/1
  Register45/1 -> Register46/1
  Register46/1 -> Register47/1
  Register47/1 -> Register48/1
  Register48/1 -> Register49/1
  Register49/1 -> Register50/1
  Register50/1 -> Register51/1
  Register51/1 -> Register52/1
  Register52/1 -> Register53/1
  Register53/1 -> Register54/1
  Register54/1 -> Register55/1
  Register55/1 -> Register56/1
  Register56/1 -> Register57/1
  Register57/1 -> Register58/1
  Register58/1 -> Register59/1
  Register59/1 -> Register60/1
  Register60/1 -> Register61/1
  Register61/1 -> Register62/1
  Register62/1 -> Register63/1
  Register63/1 -> Register64/1
  Register64/1 -> Register65/1
  Register65/1 -> Register66/1
  Register66/1 -> Register67/1
  Register67/1 -> Register68/1
  Register68/1 -> Register69/1
  Register69/1 -> Register70/1
  Register70/1 -> Register71/1
  Register71/1 -> Register72/1
  Register72/1 -> Register73/1
  Register73/1 -> Register74/1
  Register74/1 -> Register75/1
  Register75/1 -> Register76/1
  Register76/1 -> Register77/1
  Register77/1 -> Register78/1
  Register78/1 -> Register79/1
  Register79/1 -> Register80/1
  Register80/1 -> Register81/1
  Register81/1 -> Register82/1
  Register82/1 -> Register83/1
  Register83/1 -> Register84/1
  Register84/1 -> Register85/1
  Register85/1 -> Register86/1
  Register86/1 -> Register87/1
  Register87/1 -> Register88/1
  Register88/1 -> Register89/1
  Register89/1 -> Register90/1
  Register90/1 -> Register91/1
  Register91/1 -> Register92/1
  Register92/1 -> Register93/1
  Register93/1 -> Register94/1
  Register94/1 -> Register95/1
  Register95/1 -> Register96/1
  Register96/1 -> Register97/1
  Register97/1 -> Register98/1
  Register98/1 -> Register99/1
  Register99/1 -> Register100/1
  Register100/1 -> Register101/1
  Register101/1 -> Register102/1
  Register102/1 -> Register103/1
  Register103/1 -> Register104/1
  Register104/1 -> Register105/1
  Register105/1 -> Register106/1
  Register106/1 -> Register107/1
  Register107/1 -> Register108/1
  Register108/1 -> Register109/1
  Register109/1 -> Register110/1
  Register110/1 -> Register111/1
  Register111/1 -> Register112/1
  Register112/1 -> Register113/1
  Register113/1 -> Register114/1
  Register114/1 -> Register115/1
  Register115/1 -> Register116/1
  Register116/1 -> Register117/1
  Register117/1 -> Register118/1
  Register118/1 -> Register119/1
  Register119/1 -> Register120/1
  Register120/1 -> Register121/1
  Register121/1 -> Register122/1
  Register122/1 -> Register123/1
  Register123/1 -> Register124/1
  Register124/1 -> Register125/1
  Register125/1 -> Register126/1
  Register126/1 -> Register127/1
  Register127/1 -> Register128/1
  Register128/1 -> Register129/1
  Register129/1 -> Register130/1
  Register130/1 -> Register131/1
  Register131/1 -> Register132/1
  Register132/1 -> Register133/1
  Register133/1 -> Register134/1
  Register134/1 -> Register135/1
  Register135/1 -> Register136/1
  Register136/1 -> Register137/1
  Register137/1 -> Register138/1
  Register138/1 -> Register139/1
  Register139/1 -> Register140/1
  Register140/1 -> Register141/1
  Register141/1 -> Register142/1
  Register142/1 -> Register143/1
  Register143/1 -> Register144/1
  Register144/1 -> Register145/1
  Register145/1 -> Register146/1
  Register146/1 -> Register147/1
  Register147/1 -> Register148/1
  Register148/1 -> Register149/1
  Register149/1 -> Register150/1
  Register150/1 -> Register151/1
  Register151/1 -> Register152/1
  Register152/1 -> Register153/1
  Register153/1 -> Register154/1
  Register154/1 -> Register155/1
  Register155/1 -> Register156/1
  Register156/1 -> Register157/1
  Register157/1 -> Register158/1
  Register158/1 -> Register159/1
  Register159/1 -> Register160/1
  Register160/1 -> Register161/1
  Register161/1 -> Register162/1
  Register162/1 -> Register163/1
  Register163/1 -> Register164/1
  Register164/1 -> Register165/1
  Register165/1 -> Register166/1
  Register166/1 -> Register167/1
  Register167/1 -> Register168/1
  Register168/1 -> Register169/1
  Register169/1 -> Register170/1
  Register170/1 -> Register171/1
  Register171/1 -> Register172/1
  Register172/1 -> Register173/1
  Register173/1 -> Register174/1
  Register174/1 -> Register175/1
  Register175/1 -> Register176/1
  Register176/1 -> Register177/1
  Register177/1 -> Register178/1
  Register178/1 -> Register179/1
  Register179/1 -> Register180/1
  Register180/1 -> Register181/1
  Register181/1 -> Register182/1
  Register182/1 -> Register183/1
  Register183/1 -> Register184/1
  Register184/1 -> Register185/1
  Register185/1 -> Register186/1
  Register186/1 -> Register187/1
  Register187/1 -> Register188/1
  Register188/1 -> Register189/1
  Register189/1 -> Register190/1
  Register190/1 -> Register191/1
  Register191/1 -> Register192/1
  Register192/1 -> Register193/1
  Register193/1 -> Register194/1
  Register194/1 -> Register195/1
  Register195/1 -> Register196/1
  Register196/1 -> Register197/1
  Register197/1 -> Register198/1
  Register198/1 -> Register199/1
  Register199/1 -> Register200/1
  Register200/1 -> Register201/1
  Register201/1 -> Register202/1
  Register202/1 -> Register203/1
  Register203/1 -> Register204/1
  Register204/1 -> Register205/1
  Register205/1 -> Register206/1
  Register206/1 -> Register207/1
  Register207/1 -> Register208/1
  Register208/1 -> Register209/1
  Register209/1 -> Register210/1
  Register210/1 -> Register211/1
  Register211/1 -> Register212/1
  Register212/1 -> Register213/1
  Register213/1 -> Register214/1
  Register214/1 -> Register215/1
  Register215/1 -> Register216/1
  Register216/1 -> Register217/1
  Register217/1 -> Register218/1
  Register218/1 -> Register219/1
  Register219/1 -> Register220/1
  Register220/1 -> Register221/1
  Register221/1 -> Register222/1
  Register222/1 -> Register223/1
  Register223/1 -> Register224/1
  Register224/1 -> Register225/1
  Register225/1 -> Register226/1
  Register226/1 -> Register227/1
  Register227/1 -> Register228/1
  Register228/1 -> Register229/1
  Register229/1 -> Register230/1
  Register230/1 -> Register231/1
  Register231/1 -> Register232/1
  Register232/1 -> Register233/1
  Register233/1 -> Register234/1
  Register234/1 -> Register235/1
  Register235/1 -> Register236/1
  Register236/1 -> Register237/1
  Register237/1 -> Register238/1
  Register238/1 -> Register239/1
  Register239/1 -> Register240/1
  Register240/1 -> Register241/1
  Register241/1 -> Register242/1
  Register242/1 -> Register243/1
  Register243/1 -> Register244/1
  Register244/1 -> Register245/1
  Register245/1 -> Register246/1
  Register246/1 -> Register247/1
  Register247/1 -> Register248/1
  Register248/1 -> Register249/1
  d/1 -> Register0/1
  Register249/1 -> q/1

== system pfb_coeff_sim/pipeline41 ==
  d : Inport
  Register0 : xbsIndex_r4/Register  init=0  rst=off  en=off  dbl_ovrd=off  block_type=register
      settings: block_version=11.4
  Register1 : xbsIndex_r4/Register  init=0  rst=off  en=off  dbl_ovrd=off  block_type=register
      settings: block_version=11.4
  q : Outport
  wires:
  Register0/1 -> Register1/1
  d/1 -> Register0/1
  Register1/1 -> q/1

== system pfb_coeff_sim/pipeline44 ==
  d : Inport
  Register0 : xbsIndex_r4/Register  init=0  rst=off  en=off  dbl_ovrd=off  block_type=register
      settings: block_version=11.4
  Register1 : xbsIndex_r4/Register  init=0  rst=off  en=off  dbl_ovrd=off  block_type=register
      settings: block_version=11.4
  q : Outport
  wires:
  Register1/1 -> q/1
  d/1 -> Register0/1
  Register0/1 -> Register1/1

== system pfb_coeff_sim/pipeline45 ==
  d : Inport
  Register0 : xbsIndex_r4/Register  init=0  rst=off  en=off  dbl_ovrd=off  block_type=register
      settings: block_version=11.4
  Register1 : xbsIndex_r4/Register  init=0  rst=off  en=off  dbl_ovrd=off  block_type=register
      settings: block_version=11.4
  q : Outport
  wires:
  Register0/1 -> Register1/1
  d/1 -> Register0/1
  Register1/1 -> q/1

== system pfb_coeff_sim/pipeline5 ==
  d : Inport
  Register0 : xbsIndex_r4/Register  init=0  rst=off  en=off  dbl_ovrd=off  block_type=register
      settings: block_version=11.4
  Register1 : xbsIndex_r4/Register  init=0  rst=off  en=off  dbl_ovrd=off  block_type=register
      settings: block_version=11.4
  q : Outport
  wires:
  Register1/1 -> q/1
  d/1 -> Register0/1
  Register0/1 -> Register1/1

== system pfb_coeff_sim/pipeline50 ==
  d : Inport
  Register0 : xbsIndex_r4/Register  init=0  rst=off  en=off  dbl_ovrd=off  block_type=register
      settings: block_version=11.4
  Register1 : xbsIndex_r4/Register  init=0  rst=off  en=off  dbl_ovrd=off  block_type=register
      settings: block_version=11.4
  q : Outport
  wires:
  Register0/1 -> Register1/1
  d/1 -> Register0/1
  Register1/1 -> q/1

== system pfb_coeff_sim/pipeline51 ==
  d : Inport
  Register0 : xbsIndex_r4/Register  init=0  rst=off  en=off  dbl_ovrd=off  block_type=register
      settings: block_version=11.4
  Register1 : xbsIndex_r4/Register  init=0  rst=off  en=off  dbl_ovrd=off  block_type=register
      settings: block_version=11.4
  q : Outport
  wires:
  Register1/1 -> q/1
  d/1 -> Register0/1
  Register0/1 -> Register1/1

== system pfb_coeff_sim/pipeline6 ==
  d : Inport
  Register0 : xbsIndex_r4/Register  init=0  rst=off  en=off  dbl_ovrd=off  block_type=register
      settings: block_version=11.4
  Register1 : xbsIndex_r4/Register  init=0  rst=off  en=off  dbl_ovrd=off  block_type=register
      settings: block_version=11.4
  q : Outport
  wires:
  Register0/1 -> Register1/1
  d/1 -> Register0/1
  Register1/1 -> q/1

== system pfb_coeff_sim/pipeline7 ==
  d : Inport
  Register0 : xbsIndex_r4/Register  init=0  rst=off  en=off  dbl_ovrd=off  block_type=register
      settings: block_version=11.4
  Register1 : xbsIndex_r4/Register  init=0  rst=off  en=off  dbl_ovrd=off  block_type=register
      settings: block_version=11.4
  q : Outport
  wires:
  Register1/1 -> q/1
  d/1 -> Register0/1
  Register0/1 -> Register1/1
